simulink model "simple_bram_vacc_blk"  (R2019a)
settings: Solver=VariableStepAuto  StartTime=0.0  StopTime=10.0  RelTol=1e-3
libraries: xbsIndex_r4 x1
settings Model: Creator=mybur  LastModifiedBy=mybur

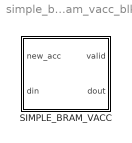
== system simple_bram_vacc_blk ==
  SIMPLE_BRAM_VACC : Subsystem  mask{vector_length=8, output_bit_w=8, output_bin_pt=0, output_sign=on}
      mask prompts: vector_length "Vector length"; output_bit_w "Bitwidth (output)"; output_bin_pt "Binary point (output)"; output_sign "Signed output?"
      mask init:
      | Simulink.Block.eval([gcb, '/simple_bram_vacc']);
      mask DialogControl DescTextVar Prompt: This simple vector accumulator is based on a shift register. It outputs its previous accumulated vector after a new_acc pulse is received.

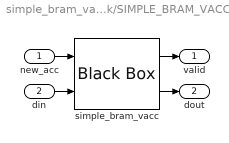
== system simple_bram_vacc_blk/SIMPLE_BRAM_VACC ==
  new_acc : Inport
  din : Inport  Port=2
  simple_bram_vacc : xbsIndex_r4/Black Box  init_code=simple_bram_vacc_config  sim_method=ISE Simulator  verbose=off  block_type=blackbox2
  valid : Outport
  dout : Outport  Port=2
  wires:
  new_acc/1 -> simple_bram_vacc/1
  simple_bram_vacc/1 -> valid/1
  din/1 -> simple_bram_vacc/2
  simple_bram_vacc/2 -> dout/1
